simulink model "fourth2nd"  (R2021b)
settings: Solver=VariableStepAuto  StartTime=1  StopTime=5  RelTol=1e-3
settings Model: Creator=minna  LastModifiedBy=minna

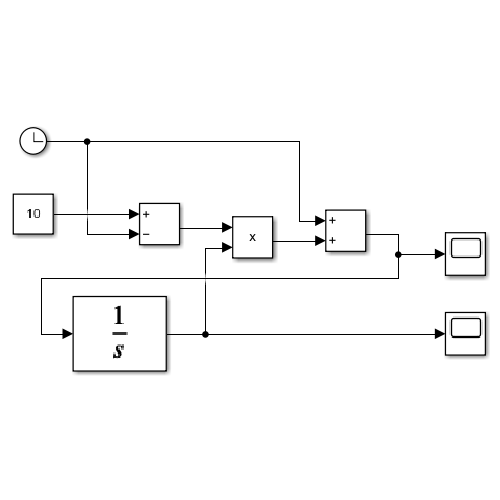
[thumbnail: Simulink's stored preview of the top-level diagram]
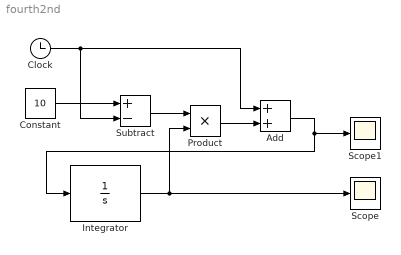
== system fourth2nd ==
  Add : Sum
  Clock : Clock
      settings: Decimation=5
  Constant : Constant  Value=10
  Integrator : Integrator  InitialCondition=1
  Product : Product
  Scope : Scope
  Scope1 : Scope
  Subtract : Sum  Inputs=+-
  wires:
  Integrator/1 -> Product/2, Scope/1
  Constant/1 -> Subtract/1
  Subtract/1 -> Product/1
  Product/1 -> Add/2
  Add/1 -> Scope1/1, Integrator/1
  Clock/1 -> Subtract/2, Add/1
